simulink model "empirical_module_hppc"  (R2024b)
settings: Solver=FixedStepAuto  StartTime=0.0  StopTime=1400  FixedStep=sim_step_time  RelTol=1e-3
PreLoadFcn:
  | open('C:\GitHub\module_ecm_analysis\empirical_module_hppc_initialisation.m');
  | run('C:\GitHub\module_ecm_analysis\empirical_module_hppc_initialisation.m');
settings Model: PacingRate=2  Creator=CARSCH  LastModifiedBy=CARSCH

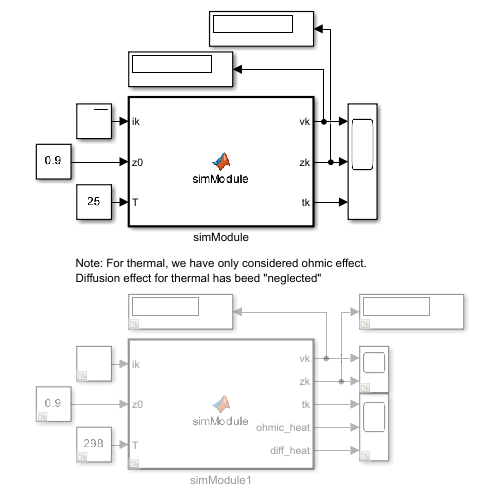
[thumbnail: Simulink's stored preview of the top-level diagram]
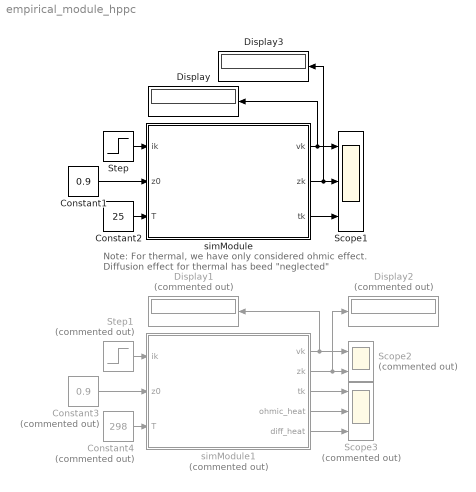
== system empirical_module_hppc ==
  note: Note: For thermal, we have only considered ohmic effect.
      | Diffusion effect for thermal has beed "neglected"
  Constant1 : Constant  Value=0.9
  Constant2 : Constant  Value=25
  Constant3 : Constant  Commented=on  Value=0.9
  Constant4 : Constant  Commented=on  Value=298
  Display : Display
  Display1 : Display  Commented=on
  Display2 : Display  Commented=on
  Display3 : Display
  Scope1 : Scope  NumInputPorts=3
  Scope2 : Scope  Commented=on  NumInputPorts=2
  Scope3 : Scope  Commented=on  NumInputPorts=3
  Step : Step  Time=5  After=300  SampleTime=0
  Step1 : Step  Commented=on  Time=5  After=300  SampleTime=0
  simModule : MATLAB Function  TreatAsAtomicUnit=on
  simModule1 : MATLAB Function  Commented=on  TreatAsAtomicUnit=on
  wires:
  Constant1/1 -> simModule/2(z0)
  Step/1 -> simModule/1(ik)
  Constant2/1 -> simModule/3(T)
  simModule/2(zk) -> Display3/1, Scope1/2
  simModule/1(vk) -> Display/1, Scope1/1
  Step1/1 -> simModule1/1(ik)
  simModule1/2(zk) -> Scope2/2, Display2/1
  Constant4/1 -> simModule1/3(T)
  simModule1/1(vk) -> Scope2/1, Display1/1
  Constant3/1 -> simModule1/2(z0)
  simModule1/5(diff_heat) -> Scope3/3
  simModule1/4(ohmic_heat) -> Scope3/2
  simModule1/3(tk) -> Scope3/1
  simModule/3(tk) -> Scope1/3

== matlab function empirical_module_hppc/simModule ==
  data: ik input; vk output; zk output; z0 input; soc_range data_store_memory; ocv_range data_store_memory; ohmic_range data_store_memory; first_pol_range data_store_memory; second_pol_range data_store_memory; first_time_range data_store_memory; second_time_range data_store_memory; deltaT data_store_memory; T input; temp_range data_store_memory; Q data_store_memory; eta data_store_memory; tk output
% function [vk,zk] = simCell(ik,z_init,temp)
% Simulates an ESC model for input current ik at temperature T
% Inputs:  ik - current, where (+) is discharge (A)
%          temp - temperature (degK)
%          z_init - initial cell state of charge (0-1)
% Outputs: vk - module resultant voltage (V)
%          zk - module state of charge (0-1)
%          tk - module thermal heat generated (i2R) (W)

% Copyright (c) 2015 by Gregory L. Plett of the University of Colorado 
% Colorado Springs (UCCS). This work is licensed under a Creative Commons 
% Attribution-NonCommercial-ShareAlike 4.0 Intl. License, v. 1.0.
% It is provided "as is", without express or implied warranty, for 
% educational and informational purposes only.
%
% This file is provided as a supplement to: Plett, Gregory L., "Battery
% Management Systems, Volume I, Battery Modeling," Artech House, 2015.

function [vk,zk,tk] = simModule(ik,z0,T) 
  global Q deltaT eta soc_range ocv_range temp_range ohmic_range... 
    first_pol_range second_pol_range first_time_range second_time_range
  persistent z_prev iR_prev;
  
  if isempty(z_prev)
    z_prev = z0;
    iR_prev = [0,0];
  end 
  
  etaik = ik; 
  % include eta in calculation for discharging current
  % includes sign of current
  etaik(ik<0) = eta*ik(ik<0); % compensate for coulombic efficiency
  if (T>40) || (T<10)
      error ('Temp Out of Range');  end

  R1C1param = interp2(temp_range, soc_range, first_time_range, T, z_prev);
  R2C2param = interp2(temp_range, soc_range, second_time_range, T, z_prev);
  RCfact = exp(-deltaT./abs([R1C1param, R2C2param]))';
  % Simulate the dynamic states of the model
  iRk = RCfact'.*iR_prev + (1-RCfact')*etaik;
  zk = z_prev - (etaik * deltaT / (Q * 3600)); 
   
  if (zk>1) || (zk<0) 
      error('SOC Out of Range'); end

  % Compute output equation
  OCV = interp2(temp_range, soc_range, ocv_range, T, zk);
  R1param = interp2(temp_range, soc_range, first_pol_range, T, zk);
  R2param = interp2(temp_range, soc_range, second_pol_range, T, zk);
  RParam = [R1param, R2param];
  R0Param = interp2(temp_range, soc_range, ohmic_range, T, zk);
  ohmic_drop = etaik*R0Param;
  diff_drop = iRk*RParam';
  vk = OCV - ohmic_drop - diff_drop;
  
  ohmic_heat = (etaik.^2)*R0Param; 
  diff_heat = 0;%(iRk.^2)*RParam';
  tk = ohmic_heat + diff_heat;

  % Update persistent variables
  z_prev = zk;
  iR_prev = iRk;

== matlab function empirical_module_hppc/simModule1 ==
  data: ik input; vk output; zk output; z0 input; soc_range data_store_memory; ocv_range data_store_memory; ohmic_range data_store_memory; first_pol_range data_store_memory; second_pol_range data_store_memory; first_time_range data_store_memory; second_time_range data_store_memory; deltaT data_store_memory; T input; temp_range data_store_memory; Q data_store_memory; eta data_store_memory; tk output; ohmic_heat output; diff_heat output
% function [vk,zk] = simCell(ik,z_init,temp)
% Simulates an ESC model for input current ik at temperature T
% Inputs:  ik - current, where (+) is discharge (A)
%          temp - temperature (degK)
%          z_init - initial cell state of charge (0-1)
% Outputs: vk - module resultant voltage (V)
%          zk - module state of charge (0-1)
%          tk - module thermal heat generated (i2R) (W)

% Copyright (c) 2015 by Gregory L. Plett of the University of Colorado 
% Colorado Springs (UCCS). This work is licensed under a Creative Commons 
% Attribution-NonCommercial-ShareAlike 4.0 Intl. License, v. 1.0.
% It is provided "as is", without express or implied warranty, for 
% educational and informational purposes only.
%
% This file is provided as a supplement to: Plett, Gregory L., "Battery
% Management Systems, Volume I, Battery Modeling," Artech House, 2015.

function [vk,zk,tk,ohmic_heat,diff_heat] = simModule(ik,z0,T) 
  global Q deltaT eta soc_range ocv_range temp_range ohmic_range... 
    first_pol_range second_pol_range first_time_range second_time_range
  persistent z_prev;
  
  if isempty(z_prev)
    z_prev = z0;
  end 
  
  etaik = ik; 
  % include eta in calculation for discharging current
  % includes sign of current
  etaik(ik<0) = eta*ik(ik<0); % compensate for coulombic efficiency
  if (T>313) || (T<283)
      error ('Temp Out of Range');  end

  R1C1param = interp2(temp_range, soc_range, first_time_range, T, z_prev);
  R2C2param = interp2(temp_range, soc_range, second_time_range, T, z_prev);
  RCfact = exp(-deltaT./abs([R1C1param, R2C2param]))';
  % Simulate the dynamic states of the model
  iRk = (1-RCfact')*etaik;
  zk = z_prev - (etaik * deltaT / (Q * 3600)); 
   
  if (zk>1) || (zk<0) 
      error('SOC Out of Range'); end

  % Compute output equation
  OCV = interp2(temp_range, soc_range, ocv_range, T, zk);
  R1param = interp2(temp_range, soc_range, first_pol_range, T, zk);
  R2param = interp2(temp_range, soc_range, second_pol_range, T, zk);
  RParam = [R1param, R2param];
  R0Param = interp2(temp_range, soc_range, ohmic_range, T, zk);
  ohmic_drop = etaik*R0Param;
  diff_drop = iRk*RParam';
  vk = OCV - ohmic_drop - diff_drop;
  
  diff_heat = (iRk.^2)*RParam';
  ohmic_heat = (etaik.^2)*R0Param;
  tk = ohmic_heat + diff_heat;

  % Update persistent variables
  z_prev = zk;
